simulink model "Mission_Server_LeaderFollower_QBot2_QDrone_FrSky"  (Simulink 9.1)
settings: Solver=ode2  StartTime=0.0  StopTime=inf  FixedStep=0.001  RelTol=1e-3  EnableMultiTasking=on
undefined symbols (not defined in the file): Host, qc_get_step_size
libraries: quarc_library x34, simulink x5
(part 2 of 2)

== system Mission_Server_LeaderFollower_QBot2_QDrone_FrSky/MISSION SERVER - LEADER/FOLLOWER with QBot 2e and QDrone/JOYSTICK/Pulse Check ==
  note: For this subsystem we will count the number of new pulses. The data can be considered enabled once the count of new signals has gone beyond 1. This will enable the Initializing and conditioning subsystem.
  new : Inport
  Compare : quarc_library/Logic Operations/Compare  operator=>=  output_data_type=boolean
      settings: SourceProductName=QUARC Targets
  Pulse Check : Constant
  "pulse count " : Subsystem  TreatAsAtomicUnit=on
  signal enable : Outport  InitialOutput=0
  wires:
  Compare/1 -> signal enable/1
  Pulse Check/1 -> Compare/2
  new/1 -> "pulse count "/Trigger
  "pulse count "/1(Number of Pulses) -> Compare/1

== system Mission_Server_LeaderFollower_QBot2_QDrone_FrSky/MISSION SERVER - LEADER/FOLLOWER with QBot 2e and QDrone/Data Server (Localization) /Convention Correction (Motive Frame to Research Studio Frame) - QBot 2e/Prevent Gimbal Lock ==
  note: Remapping the rotation order to prevent gimbal lock
      | in heading/yaw due to Euler singularity condition
  Attitude (rad) [3] : Inport
  Demux : Demux  Outputs=3
  Euler Angles from Rotation Matrix (Relative ZYX) : quarc_library/Math Operations/Matrices/Euler Angles from Rotation Matrix  menu_order=Relative Z-Y-X
      settings: SourceProductName=QUARC Targets
  Euler Angles to Rotation Matrix (Relative YZX) : quarc_library/Math Operations/Matrices/Euler Angles to Rotation Matrix  menu_order=Relative Y-Z-X
      settings: SourceProductName=QUARC Targets
  Mux : Mux  Inputs=3
  "Attitude (rad) [3] " : Outport
  wires:
  Demux/1 -> Euler Angles to Rotation Matrix (Relative YZX)/3
  Demux/3 -> Euler Angles to Rotation Matrix (Relative YZX)/2
  Demux/2 -> Euler Angles to Rotation Matrix (Relative YZX)/1
  Mux/1 -> "Attitude (rad) [3] "/1
  Attitude (rad) [3]/1 -> Demux/1
  Euler Angles to Rotation Matrix (Relative YZX)/1 -> Euler Angles from Rotation Matrix (Relative ZYX)/1
  Euler Angles from Rotation Matrix (Relative ZYX)/3 -> Mux/1
  Euler Angles from Rotation Matrix (Relative ZYX)/1 -> Mux/3
  Euler Angles from Rotation Matrix (Relative ZYX)/2 -> Mux/2

== system Mission_Server_LeaderFollower_QBot2_QDrone_FrSky/MISSION SERVER - LEADER/FOLLOWER with QBot 2e and QDrone/Data Server (Localization) /Convention Correction  (Motive Frame to Research Studio Frame) - QDrone/Prevent Gimbal Lock ==
  note: Remapping the rotation order to prevent gimbal lock
      | in heading/yaw due to Euler singularity condition
  Attitude (rad) [3] : Inport
  Demux : Demux  Outputs=3
  Euler Angles from Rotation Matrix (Relative ZYX) : quarc_library/Math Operations/Matrices/Euler Angles from Rotation Matrix  menu_order=Relative Z-Y-X
      settings: SourceProductName=QUARC Targets
  Euler Angles to Rotation Matrix (Relative YZX) : quarc_library/Math Operations/Matrices/Euler Angles to Rotation Matrix  menu_order=Relative Y-Z-X
      settings: SourceProductName=QUARC Targets
  Mux : Mux  Inputs=3
  "Attitude (rad) [3] " : Outport
  wires:
  Demux/1 -> Euler Angles to Rotation Matrix (Relative YZX)/3
  Demux/3 -> Euler Angles to Rotation Matrix (Relative YZX)/2
  Demux/2 -> Euler Angles to Rotation Matrix (Relative YZX)/1
  Mux/1 -> "Attitude (rad) [3] "/1
  Attitude (rad) [3]/1 -> Demux/1
  Euler Angles to Rotation Matrix (Relative YZX)/1 -> Euler Angles from Rotation Matrix (Relative ZYX)/1
  Euler Angles from Rotation Matrix (Relative ZYX)/3 -> Mux/1
  Euler Angles from Rotation Matrix (Relative ZYX)/1 -> Mux/3
  Euler Angles from Rotation Matrix (Relative ZYX)/2 -> Mux/2

== system Mission_Server_LeaderFollower_QBot2_QDrone_FrSky/MISSION SERVER - LEADER/FOLLOWER with QBot 2e and QDrone/JOYSTICK/Pulse Check/pulse count  ==
  Trigger : TriggerPort  TriggerType=either  VariantControl=Variant
  Constant1 : Constant  Value=0
  Increment Stored Integer : simulink/Additional Math & Discrete/Additional Math: Increment - Decrement/Increment Stored Integer
  Sum : Sum  Inputs=|++
  Unit Delay : UnitDelay  SampleTime=-1
  Number of Pulses : Outport
  wires:
  Constant1/1 -> Sum/1
  Sum/1 -> Increment Stored Integer/1
  Unit Delay/1 -> Sum/2
  Increment Stored Integer/1 -> Unit Delay/1, Number of Pulses/1

== matlab function MISSION SERVER - LEADER//FOLLOWER with QBot 2e and QDrone/Extract Vehicle Data - QBot 2e/Extract Object Data ==
  data: data input double; position output double; orientation output double; index input double; tracking output double
function [position, orientation, tracking] = fcn(data, index)

n = length(data)/7;

if (index<=0)||(index>n)
    position = zeros(1,3); orientation = zeros(1,3); tracking = 0;
else
    position = [data(index*3-2), data(index*3-1), data(index*3)];
    orientation = [data((index+n)*3 - 2), data((index+n)*3 - 1), data((index+n)*3)];
    tracking = data(index + (n*6));
end

== matlab function MISSION SERVER - LEADER//FOLLOWER with QBot 2e and QDrone/Extract Vehicle Data - QDrone/Extract Object Data ==
  data: data input double; position output double; orientation output double; index input double; tracking output double
function [position, orientation, tracking] = fcn(data, index)

n = length(data)/7;

if (index<=0)||(index>n)
    position = zeros(1,3); orientation = zeros(1,3); tracking = 0;
else
    position = [data(index*3-2), data(index*3-1), data(index*3)];
    orientation = [data((index+n)*3 - 2), data((index+n)*3 - 1), data((index+n)*3)];
    tracking = data(index + (n*6));
end

== matlab function Communication - QDrone/Detect Communication loss/MATLAB Function ==
  data: time input double; stream_connection_loss output double; state input double; error input double
function stream_connection_loss  = fcn(time, state, error)

stream_connection_loss = 0;
if time > 1
    if ~((state == 2)&&(error >= 0))
        % stream connection is not established correctly
        stream_connection_loss = 1;
    end
end

== matlab function Communication - QBot 2e/Detect Communication loss/MATLAB Function ==
  data: time input double; stream_connection_loss output double; state input double; error input double
function stream_connection_loss  = fcn(time, state, error)

stream_connection_loss = 0;
if time > 1
    if ~((state == 2)&&(error >= 0))
        % stream connection is not established correctly
        stream_connection_loss = 1;
    end
end

== matlab function MISSION SERVER - LEADER//FOLLOWER with QBot 2e and QDrone/Waypoint Scheduler/MATLAB Function1 ==
  data: x_lead input double; y_lead input double; x_ref input double; y_ref input double; z_quad input double; start_stop input double; x_cmd_ref output double; y_cmd_ref output double; status output double

function [x_cmd_ref, y_cmd_ref, status] = ...
    StateMachine(x_lead,y_lead,x_ref,y_ref,z_quad,start_stop)

persistent pre_start_stop;
persistent state;

MIN_QUAD_HEIGHT = 0.5;  % m

if( isempty(pre_start_stop) )
    pre_start_stop = start_stop;
end

if( isempty(state) )
    state = 0;  % IDLE
end

if( pre_start_stop ~= start_stop )
    hasChanged = 1;
else
    hasChanged = 0;
end

switch state
    case 0
        % IDLE state, do nothing
        x_cmd_ref = x_lead;
        y_cmd_ref = y_lead;
        status = state;
        if( hasChanged == 1 )
            % Transition to TAKEOFF state
            state = 1;
        end
    case 1
        % TAKEOFF state
        x_cmd_ref = x_lead;
        y_cmd_ref = y_lead;
        status = state;
        if( z_quad >= MIN_QUAD_HEIGHT )
            % Transition to WAYPOINT state
            state = 2;
        elseif( hasChanged == 1 )
            % Transition to LANDING state
            state = 3;
            status = state;
        end
    case 2
        % WAYPOINT state - passing through waypoints
        x_cmd_ref = x_ref;
        y_cmd_ref = y_ref;
        status = state;
        if( hasChanged == 1 )
            % Transition to LANDING state
            state = 3;
            status = state;
        end
    case 3
        % LANDING state
        x_cmd_ref = x_lead;
        y_cmd_ref = y_lead;
        status = state;
    otherwise
        % ERROR State, do nothing
        x_cmd_ref = x_lead;
        y_cmd_ref = y_lead;
        status = state;
end

% Save the start_stop signal for next loop
pre_start_stop = start_stop;

== matlab function MISSION SERVER - LEADER//FOLLOWER with QBot 2e and QDrone/Waypoint Scheduler/MATLAB Function ==
  data: Arrived input double; idx output double; n input double; x_waypoints input double; y_waypoints input double; done output double; x_ref output double; y_ref output double; last_waypoint output double
function [idx, done, x_ref, y_ref, last_waypoint] = ...
    SchedulerLogic(Arrived, n, x_waypoints, y_waypoints)

persistent curr_idx;
persistent idx_incremented; 

if( isempty( curr_idx ) )
    curr_idx = 1;
end

if( isempty( idx_incremented) )
    idx_incremented = 0;
end


idx = curr_idx;
x_ref = x_waypoints(idx);
y_ref = y_waypoints(idx);
done = 0;
last_waypoint = 0;

if( Arrived == 1 ) 
    if( curr_idx == n )
        % Done
        last_waypoint = 1;
        done = 1;
    else
        if( idx_incremented == 1)
            idx_incremented = 0;
        else 
        curr_idx = curr_idx + 1;        
        idx_incremented = 1;
        end 
    end
else 
    idx_incremented = 0;
end
